simulink model "Sim_Non_linear_Model_Twin_Engine_UAV"  (Simulink 7.7)
settings: Solver=ode45  StartTime=0.0  StopTime=100  RelTol=1e-3
values from neighbouring files (symbols this model uses):
  b = 11.02    [Nonlinear_Simulation_Twin_Engine_Data.m]
  C = 2    [Nonlinear_Simulation_Twin_Engine_Data.m]
  c1 = [(Iy-Iz)*Iz-Ixz^2]/G    [Nonlinear_Simulation_Twin_Engine_Data.m]
  c2 = [(Ix-Iy+Iz)*Ixz]/G    [Nonlinear_Simulation_Twin_Engine_Data.m]
  c3 = Iz/G    (= 0.108008192931)    [Nonlinear_Simulation_Twin_Engine_Data.m]
  c4 = Ixz/G    (= 0.00967627878562)    [Nonlinear_Simulation_Twin_Engine_Data.m]
  c5 = (Iz-Ix)/Iy    (= 0.566728971963)    [Nonlinear_Simulation_Twin_Engine_Data.m]
  c6 = Ixz/Iy    (= 0.207476635514)    [Nonlinear_Simulation_Twin_Engine_Data.m]
  c7 = 1/Iy    (= 0.18691588785)    [Nonlinear_Simulation_Twin_Engine_Data.m]
  c8 = [Ix*(Ix-Iy)+Ixz^2]/G    [Nonlinear_Simulation_Twin_Engine_Data.m]
  c9 = Ix/G    (= 0.0815771323206)    [Nonlinear_Simulation_Twin_Engine_Data.m]
  cbar = C    (= 2)    [Nonlinear_Simulation_Twin_Engine_Data.m]
  CDa = 0.149    [Nonlinear_Simulation_Twin_Engine_Data.m]
  CDad = 0    [Nonlinear_Simulation_Twin_Engine_Data.m]
  CDde = 0.0363    [Nonlinear_Simulation_Twin_Engine_Data.m]
  CDo = 0.032    [Nonlinear_Simulation_Twin_Engine_Data.m]
  CDq = 0.0    (= 0)    [Nonlinear_Simulation_Twin_Engine_Data.m]
  CDu = 0    [Nonlinear_Simulation_Twin_Engine_Data.m]
  CLa = 4.817    [Nonlinear_Simulation_Twin_Engine_Data.m]
  CLad = 2.647    [Nonlinear_Simulation_Twin_Engine_Data.m]
  Clb = -0.0717    [Nonlinear_Simulation_Twin_Engine_Data.m]
  Clda = 0.284552    [Nonlinear_Simulation_Twin_Engine_Data.m]
  CLde = 0.86    [Nonlinear_Simulation_Twin_Engine_Data.m]
  Cldr = 0.0095    [Nonlinear_Simulation_Twin_Engine_Data.m]
  CLo = 0.522    [Nonlinear_Simulation_Twin_Engine_Data.m]
  Clp = -0.4164    [Nonlinear_Simulation_Twin_Engine_Data.m]
  CLq = 6.034    [Nonlinear_Simulation_Twin_Engine_Data.m]
  Clr = 0.1393    [Nonlinear_Simulation_Twin_Engine_Data.m]
  CLu = .005    (= 0.005)    [Nonlinear_Simulation_Twin_Engine_Data.m]
  Cma = -.963    (= -0.963)    [Nonlinear_Simulation_Twin_Engine_Data.m]
  Cmad = -9.9    [Nonlinear_Simulation_Twin_Engine_Data.m]
  Cmde = -1.467167    [Nonlinear_Simulation_Twin_Engine_Data.m]
  Cmo = -0.17    [Nonlinear_Simulation_Twin_Engine_Data.m]
  Cmq = -7.225    [Nonlinear_Simulation_Twin_Engine_Data.m]
  Cmu = .00028    (= 0.00028)    [Nonlinear_Simulation_Twin_Engine_Data.m]
  Cnb = 0.062324    [Nonlinear_Simulation_Twin_Engine_Data.m]
  Cnda = 0    [Nonlinear_Simulation_Twin_Engine_Data.m]
  Cndr = -0.066583    [Nonlinear_Simulation_Twin_Engine_Data.m]
  Cnp = -0.032818    [Nonlinear_Simulation_Twin_Engine_Data.m]
  Cnr = -0.094971    [Nonlinear_Simulation_Twin_Engine_Data.m]
  Cyb = -0.26557    [Nonlinear_Simulation_Twin_Engine_Data.m]
  Cyda = 0.0    (= 0)    [Nonlinear_Simulation_Twin_Engine_Data.m]
  Cydr = 0.145141    [Nonlinear_Simulation_Twin_Engine_Data.m]
  Cyp = -0.121995    [Nonlinear_Simulation_Twin_Engine_Data.m]
  Cyr = 0.12987    [Nonlinear_Simulation_Twin_Engine_Data.m]
  g = 32.2    [Nonlinear_Simulation_Twin_Engine_Data.m]
  m = W/g    (= 2.17391304348)    [Nonlinear_Simulation_Twin_Engine_Data.m]
  qbar = q1    [Nonlinear_Simulation_Twin_Engine_Data.m]
  ro = 0.00215213    [Nonlinear_Simulation_Twin_Engine_Data.m]
  S = 22.146    [Nonlinear_Simulation_Twin_Engine_Data.m]
  U0 = Vto    [Nonlinear_Simulation_Twin_Engine_Data.m]
  Vto = sqrt(uo^2+vo^2+wo^2)    [Nonlinear_Simulation_Twin_Engine_Data.m]
settings Model: Creator=nigampatel  LastModifiedBy=sbhandari

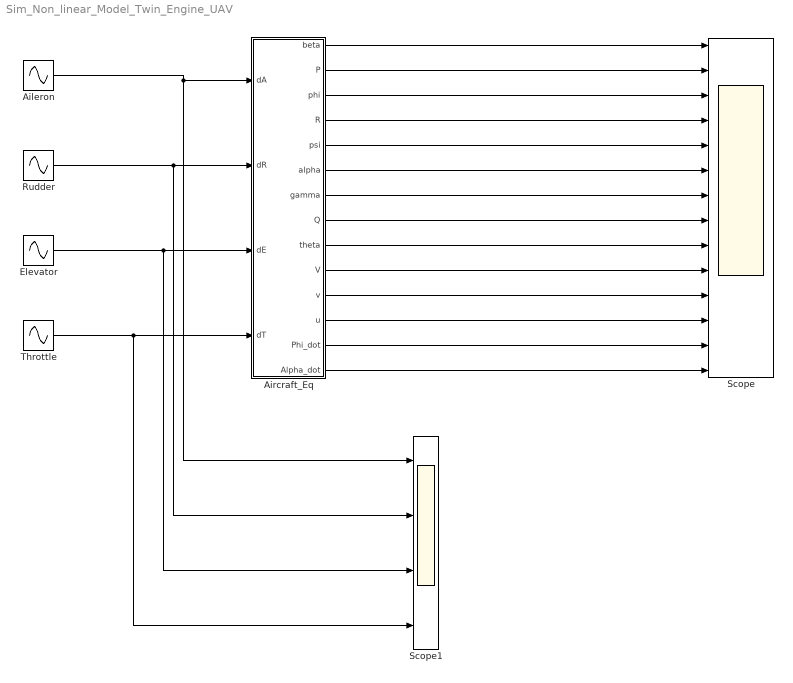
== system Sim_Non_linear_Model_Twin_Engine_UAV ==
  Aileron : Sin  Amplitude=5/57.3  Frequency=2  SampleTime=0
  Aircraft_Eq : Subsystem
  Elevator : Sin  Amplitude=0  Frequency=2  SampleTime=0
  Rudder : Sin  Amplitude=0  Frequency=2  SampleTime=0
  Scope : Scope  NumInputPorts=14
      settings: YMin=-24500~-30725~-5~-5~-5~-5~-5~-5~-5~-5~-5~-5~-5~-5  YMax=-21000~-30375~5~5~5~5~5~5~5~5~5~5~5~5
  Scope1 : Scope  NumInputPorts=4
      settings: YMin=-2.25~-2~-0.1~0.95  YMax=0.5~0.25~0.6~1.05  SaveName=ScopeData4
  Throttle : Sin  Amplitude=0  Frequency=2  SampleTime=0
  wires:
  Throttle/1 -> Scope1/4, Aircraft_Eq/4(dT)
  Elevator/1 -> Scope1/3, Aircraft_Eq/3(dE)
  Aileron/1 -> Scope1/1, Aircraft_Eq/1(dA)
  Aircraft_Eq/1(beta) -> Scope/1
  Aircraft_Eq/2(P) -> Scope/2
  Aircraft_Eq/3(phi) -> Scope/3
  Aircraft_Eq/4(R) -> Scope/4
  Aircraft_Eq/5(psi) -> Scope/5
  Aircraft_Eq/6(alpha) -> Scope/6
  Aircraft_Eq/7(gamma) -> Scope/7
  Aircraft_Eq/8(Q) -> Scope/8
  Aircraft_Eq/9(theta) -> Scope/9
  Aircraft_Eq/10(V) -> Scope/10
  Aircraft_Eq/11(v) -> Scope/11
  Aircraft_Eq/12(u) -> Scope/12
  Aircraft_Eq/13(Phi_dot) -> Scope/13
  Aircraft_Eq/14(Alpha_dot) -> Scope/14
  Rudder/1 -> Scope1/2, Aircraft_Eq/2(dR)

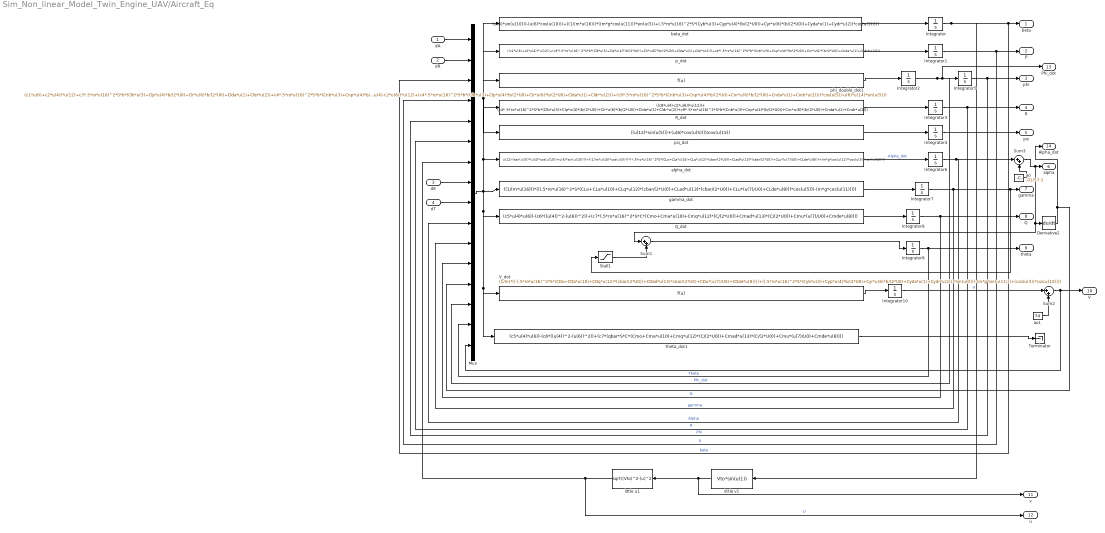
== system Sim_Non_linear_Model_Twin_Engine_UAV/Aircraft_Eq ==
  dA : Inport
  dR : Inport  Port=2
  dE : Inport  Port=3
  dT : Inport  Port=4
  Derivative2 : Derivative
  Integrator{,1..10} (11 alike) : Integrator
  Mux : Mux  Inputs=16
  Q_dot : Fcn  Expr=(c5*u(4)*u(6))-(c6*((u(4))^2-(u(6))^2))+(c7*(.5*ro*u(16)^2*S*C*(Cmo+Cma*u(10)+Cmq*u(12)*(C/(2*U0))+Cmad*u(13)*(C/(2*U0))+Cmu*(u(7)/U0)+Cmde*u(8))))
  R_dot : Fcn  Expr=((c8*u(4)-c2*u(6))*u(12))+ (c4*.5*ro*u(16)^2*S*b*(Clb*u(3)+Clp*u(4)*(b/(2*U0))+Clr*u(6)*(b/(2*U0))+Clda*u(1)+Cldr*u(2))+c9*.5*ro*u(16)^2*S*b*(Cnb*u(3)+Cnp*u(4)*(b/(2*U0))+Cnr*u(6)*(b/(2*U0))+Cnda*u(1)+Cndr*u(2)))
  Stall1 : Saturate  UpperLimit=50/57.3  LowerLimit=-50/57.3
  Sum1 : Sum  Inputs=|++  SaturateOnIntegerOverflow=on  InputSameDT=on  OutDataTypeStr=Inherit: Same as first input
  Sum2 : Sum  Inputs=|++  SaturateOnIntegerOverflow=on  InputSameDT=on  OutDataTypeStr=Inherit: Same as first input
  Sum3 : Sum  Inputs=|++  SaturateOnIntegerOverflow=on  InputSameDT=on  OutDataTypeStr=Inherit: Same as first input
  Terminator : Terminator
  V_dot : Fcn  Expr=(1/m)*((-(.5*ro*u(16)^2*S*(CDo+CDa*u(10)+CDq*u(12)*(cbar/(2*U0))+CDad*u(13)*cbar/(2*U0)+CDu*(u(7)/U0)+CDde*u(8))))+((.5*ro*u(16)^2*S*(Cyb*u(3)+Cyp*u(4)*b/(2*U0)+Cyr*u(6)*b/(2*U0)+Cyda*u(1)+Cydr*u(2)))*sin(u(3)))-(m*g*sin(u(11)))+(cos(u(3))*cos(u(10))))
  alpha_dot : Fcn  Expr=u(12)-(tan(u(3))*(u(4)*cos(u(10))+u(6)*sin(u(10))))+((1/(m*u(16)*cos(u(3))))*(-(.5*ro*u(16)^2*S*(CLo+CLa*u(10)+CLq*u(12)*(cbar/(2*U0))+CLad*u(13)*(cbar/(2*U0))+CLu*(u(7)/U0)+CLde*u(8)))+(m*g*cos(u(11))*cos(u(5)))-sin(u(10))))
  ao : Constant  Value=.01/57.3
  ao1 : Constant  Value=74
  beta_dot : Fcn  Expr=(u(4)*sin(u(10)))-(u(6)*cos(u(10)))+((1/(m*u(16)))*((m*g*cos(u(11)))*sin(u(5))+(.5*ro*u(16)^2*S*(Cyb*u(3)+Cyp*u(4)*(b/(2*U0))+Cyr*u(6)*(b/(2*U0))+Cyda*u(1)+Cydr*u(2))*cos(u(3)))))
  gamma_dot : Fcn  Expr=((1/(m*u(16)))*(((.5*ro*u(16)^2*S*(CLo+CLa*u(10)+CLq*u(12)*(cbar/(2*U0))+CLad*u(13)*(cbar/(2*U0))+CLu*(u(7)/U0)+CLde*u(8)))*cos(u(5)))-(m*g*cos(u(11)))))
  little u1 : Fcn  Expr=sqrt((Vto)^2-(u)^2)
  little v1 : Fcn  Expr=Vto*sin(u(1))
  p_dot : Fcn  Expr=((c1*u(6)+c2*u(4))*u(12))+(c3*(.5*ro*u(16)^2*S*b*(Clb*u(3)+Clp*u(4)*(b/(2*U0))+Clr*u(6)*(b/(2*U0))+Clda*u(1)+Cldr*u(2)))+c4*(.5*ro*u(16)^2*S*b*(Cnb*u(3)+Cnp*u(4)*(b/(2*U0))+Cnr*u(6)*(b/(2*U0))+Cnda*u(1)+Cndr*u(2))))
  phi_double_dot1 : Fcn  Expr=(c1*u(6)+c2*u(4))*u(12)+c3*.5*ro*u(16)^2*S*b*(Clb*u(3)+Clp*u(4)*b/(2*U0)+Clr*u(6)*b/(2*U0)+Clda*u(1)+Cldr*u(2))+c4*.5*ro*u(16)^2*S*b*(Cnb*u(3)+Cnp*u(4)*b/(2*U0)+Cnr*u(6)*b/(2*U0)+Cnda*u(1)+Cndr*u(2))+tan(u(15))*(u(12)*u(14)*cos(u(5))+((c8*u(4)-c2*u(6))*u(12)+(c4*.5*ro*u(16)^2*S*b*(Clb*u(3)+Clp*u(4)*b/(2*U0)+Clr*u(6)*b/(2*U0)+Clda*u(1)+Cldr*u(2)))+(c9*.5*ro*u(16)^2*S*b*(Cnb*u(3)+Cnp*u(4)*b/(2*U0)+Cnr*u(6)*b/(2*U0)+Cnda*u(1)+Cndr*u(2))))*cos(u(5))-u(6)*u(14)*sin(u(5)))
  psi_dot : Fcn  Expr=((u(12)*sin(u(5)))+(u(6)*cos(u(5))))/cos(u(15))
  theta_dot1 : Fcn  Expr=(c5*u(4)*u(6))-(c6*((u(4))^2-(u(6))^2))+(c7*(qbar*S*C*(Cmo+Cma*u(10)+Cmq*u(12)*(C/(2*U0))+Cmad*u(13)*(C/(2*U0))+Cmu*(u(7)/U0)+Cmde*u(8))))
  beta : Outport
  P : Outport  Port=2
  phi : Outport  Port=3
  R : Outport  Port=4
  psi : Outport  Port=5
  alpha : Outport  Port=6
  gamma : Outport  Port=7
  Q : Outport  Port=8
  theta : Outport  Port=9
  V : Outport  Port=10
  v : Outport  Port=11
  u : Outport  Port=12
  Phi_dot : Outport  Port=13
  Alpha_dot : Outport  Port=14
  wires:
  little v1/1 -> little u1/1, v/1
  Mux/1 -> beta_dot/1, phi_double_dot1/1, psi_dot/1, p_dot/1, R_dot/1, alpha_dot/1, gamma_dot/1, Q_dot/1, V_dot/1, theta_dot1/1
  little u1/1 -> Mux/7, u/1  "U"
  psi_dot/1 -> Integrator4/1
  R_dot/1 -> Integrator3/1
  phi_double_dot1/1 -> Integrator2/1
  p_dot/1 -> Integrator1/1
  beta_dot/1 -> Integrator/1
  Integrator2/1 -> Integrator5/1, Mux/14, Phi_dot/1  "Phi_dot"
  Integrator5/1 -> phi/1, Mux/5  "Phi"
  Integrator1/1 -> P/1, Mux/4  "P"
  Integrator/1 -> little v1/1, beta/1, Mux/3  "beta"
  Integrator3/1 -> R/1, Mux/6  "R"
  Integrator4/1 -> psi/1
  dR/1 -> Mux/2
  dA/1 -> Mux/1
  dE/1 -> Mux/8
  dT/1 -> Mux/9
  alpha_dot/1 -> Integrator6/1  "Alpha_dot"
  Integrator6/1 -> Mux/10, Sum3/1  "Alpha"
  gamma_dot/1 -> Integrator7/1
  Integrator7/1 -> Mux/11, gamma/1, Stall1/1  "gamma"
  Q_dot/1 -> Integrator8/1
  Integrator8/1 -> Q/1, Mux/12  "Q"
  Integrator9/1 -> theta/1, Mux/15  "Theta"
  V_dot/1 -> Integrator10/1
  ao/1 -> Sum3/2
  Sum3/1 -> alpha/1, Sum1/1, Derivative2/1
  Stall1/1 -> Sum1/2
  Sum1/1 -> Integrator9/1
  theta_dot1/1 -> Terminator/1
  Derivative2/1 -> Alpha_dot/1, Mux/13
  Integrator10/1 -> Sum2/1  "V"
  Sum2/1 -> V/1, Mux/16
  ao1/1 -> Sum2/2
